simulink model "aero_ground_model"  (R2013b)
settings: Solver=ode23  StartTime=0.0  StopTime=100  FixedStep=0.01  MaxStep=1  RelTol=1e-3
undefined symbols (not defined in the file or in its folder): par
libraries: simulink x12, coeffs x3, lateral_model x3, dspswit3 x1
(part 1 of 2)
settings Model: Creator=goghino  LastModifiedBy=Juraj
settings SolverCC: ZeroCrossAlgorithm=Adaptive  AlgebraicLoopSolver=LineSearch
settings DataIOCC: SignalLoggingSaveFormat=ModelDataLogs
settings DebuggingCC: UnderspecifiedInitializationDetection=Simplified  MultiTaskDSMMsg=warning  MultiTaskCondExecSysMsg=none  SignalLabelMismatchMsg=warning  StrictBusMsg=WarnOnBusTreatedAsVector  NonBusSignalsTreatedAsBus=warning
settings RTWCC: IncludeERTFirstTime=on
settings GRTTargetCC: CodeReplacementLibrary=None  CPPClassGenCompliant=on

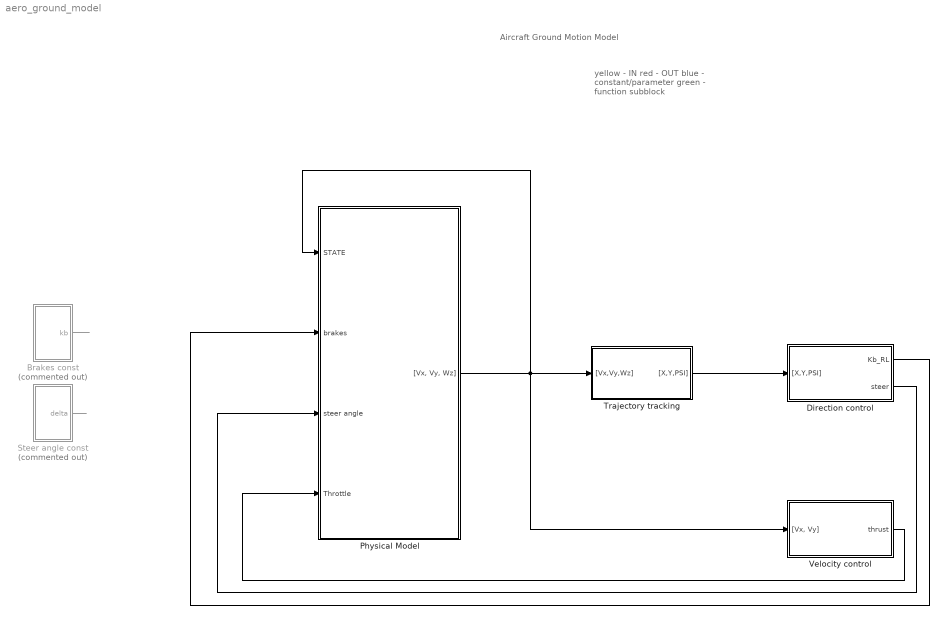
== system aero_ground_model ==
  note: Aircraft Ground Motion Model
  note: yellow - IN
      | red - OUT
      | blue - constant/parameter
      | green - function subblock
  Brakes const : Subsystem  Commented=on
  Direction control : Subsystem
  Physical Model : Subsystem
  Steer angle const : Subsystem  Commented=on
  Trajectory tracking : Subsystem
  Velocity control : Subsystem
  wires:
  Physical Model/1("[Vx, Vy, Wz]") -> Physical Model/1(STATE), Trajectory tracking/1("[Vx,Vy,Wz]"), Velocity control/1("[Vx, Vy]")
  Trajectory tracking/1("[X,Y,PSI]") -> Direction control/1("[X,Y,PSI]")
  Velocity control/1(thrust) -> Physical Model/4(Throttle)
  Direction control/2(steer) -> Physical Model/3(steer angle)
  Direction control/1(Kb_RL) -> Physical Model/2(brakes)
  Steer angle const/1(delta) -> ?
  Brakes const/1(kb) -> ?

== system aero_ground_model/Brakes const ==
  Bus Creator : BusCreator  Inputs=2
  L : Constant  Value=par.kbl
  R : Constant  Value=par.kbr
  kb : Outport
  wires:
  Bus Creator/1 -> kb/1  "Kb"
  R/1 -> Bus Creator/1  "kb_R"
  L/1 -> Bus Creator/2  "kb_L"

== system aero_ground_model/Direction control ==
  "[X,Y,PSI]" : Inport
  Bus Selector : BusSelector  OutputSignals=X,Y,PSI
  Steer PIDs : Subsystem
  Target selector : Subsystem
  To Workspace : ToWorkspace  VariableName=X  SampleTime=-1  SaveFormat=Timeseries
  To Workspace1 : ToWorkspace  VariableName=Y  SampleTime=-1  SaveFormat=Timeseries
  To Workspace2 : ToWorkspace  VariableName=PSI  SampleTime=-1  SaveFormat=Timeseries
  delta heading to target : Subsystem
  Kb_RL : Outport
  steer : Outport  Port=2
  wires:
  Bus Selector/1 -> To Workspace/1  "<X>"
  Bus Selector/2 -> To Workspace1/1  "<Y>"
  Bus Selector/3 -> To Workspace2/1  "<PSI>"
  "[X,Y,PSI]"/1 -> delta heading to target/2(Pos Aero), Target selector/1(Pos Aero), Bus Selector/1
  delta heading to target/1(heading diff) -> Steer PIDs/1("delta heading ")
  Steer PIDs/1(Kb) -> Kb_RL/1
  Steer PIDs/2(steer) -> steer/1
  Target selector/1(Target) -> delta heading to target/1(Pos Target)

== system aero_ground_model/Physical Model ==
  note: Transformation of Forces Acting on Aircraft into State Vector
  note: Physical Model of Aircraft Ground Motion Model
  STATE : Inport
  brakes : Inport  Port=2
  steer angle : Inport  Port=3
  Throttle : Inport  Port=4
  Bus Creator : BusCreator
  Bus Creator1 : BusCreator  Inputs=2
  Bus Creator3 : BusCreator  Inputs=3
  Drag : Subsystem
  Engine model : Subsystem
  Forces to Velocities : Subsystem
  Tire Forces : Subsystem
  X TIRE_FORCES : Scope
      settings: YMin=-140000  YMax=10000  SaveName=ScopeData3
  Y TIRE_FORCES1 : Scope
      settings: YMin=-140000  YMax=10000  SaveName=ScopeData4
  "[Vx, Vy, Wz]" : Outport
  wires:
  Forces to Velocities/2(angular) -> Bus Creator1/2  "Wz"
  Throttle/1 -> Engine model/1(Throttle)
  Bus Creator1/1 -> "[Vx, Vy, Wz]"/1  "STATE"
  steer angle/1 -> Tire Forces/3(delta), Forces to Velocities/8(delta)
  Drag/1(F_xA) -> Forces to Velocities/9(F_xA)
  STATE/1 -> Tire Forces/2(state), Drag/1(STATE), Forces to Velocities/10(STATE)
  Tire Forces/1(F_xN) -> Forces to Velocities/2(F_xN), Bus Creator/1
  Tire Forces/2(F_xL) -> Forces to Velocities/3(F_xL), Bus Creator/2
  Tire Forces/3(F_xR) -> Forces to Velocities/4(F_xR), Bus Creator/3
  Tire Forces/4(F_yN) -> Forces to Velocities/5(F_yN), Bus Creator3/3
  Tire Forces/5(F_yL) -> Bus Creator3/2, Forces to Velocities/6(F_yL)
  Tire Forces/6(F_yR) -> Bus Creator3/1, Forces to Velocities/7(F_yR)
  Forces to Velocities/1(velocity) -> Bus Creator1/1  "[Vx, Vy]"
  brakes/1 -> Tire Forces/4(brakes)
  Bus Creator/1 -> X TIRE_FORCES/1
  Bus Creator3/1 -> Y TIRE_FORCES1/1
  Engine model/1(F_xT) -> Tire Forces/1(thrust), Forces to Velocities/1(F_xT), Bus Creator/4

== system aero_ground_model/Steer angle const ==
  11.5 deg : Constant  Value=0.2
  20 deg : Constant  Value=0.35
  40 deg : Constant  Value=0.7
  5.7 deg : Constant  Value=0.1
  60 deg1 : Constant  Value=1.04
  90 deg : Constant  Value=1.57
  zero : Constant  Value=0
  delta : Outport
  wires:
  11.5 deg/1 -> delta/1

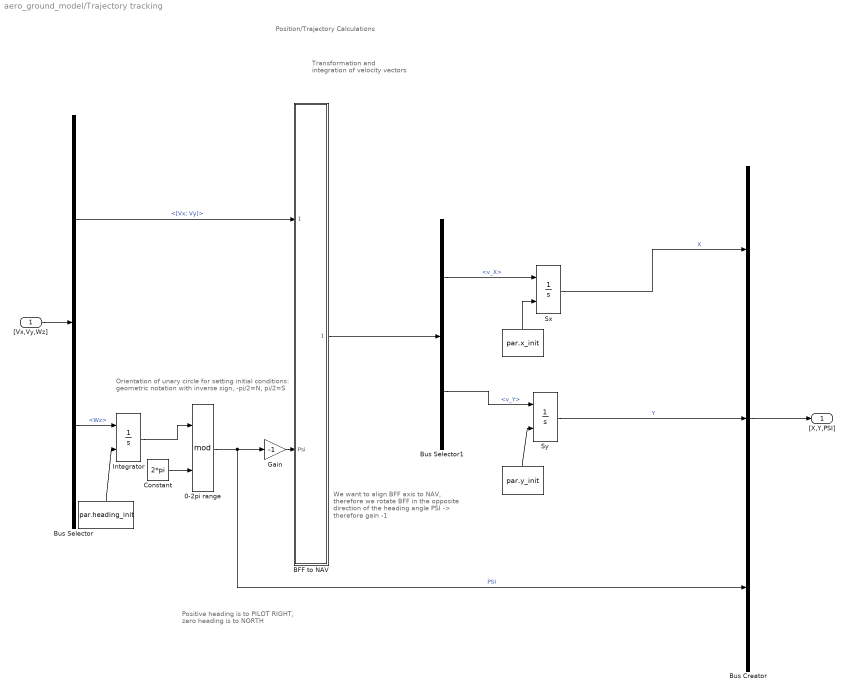
== system aero_ground_model/Trajectory tracking ==
  note: Orientation of unary circle for setting initial conditions:
      | geometric notation with inverse sign, -pi/2=N, pi/2=S
  note: Positive heading is to PILOT RIGHT,
      | zero heading is to NORTH
  note: We want to align BFF axis to NAV,
      | therefore we rotate BFF in the opposite
      | direction of the heading angle PSI ->
      | therefore gain -1
  note: Transformation and integration of velocity vectors
  note: Position/Trajectory Calculations
  "[Vx,Vy,Wz]" : Inport
  " " : Constant  Value=par.heading_init
  "   " : Constant  Value=par.y_init
  "    " : Constant  Value=par.x_init
  0-2pi range : Math  Operator=mod  SaturateOnIntegerOverflow=on
  BFF to NAV : Subsystem
  Bus Creator : BusCreator  Inputs=3
  Bus Selector : BusSelector  OutputSignals=[Vx; Vy],Wz
  Bus Selector1 : BusSelector  OutputSignals=v_X,v_Y
  Constant : Constant  Value=2*pi
  Gain : Gain  Gain=-1
  Integrator : Integrator  InitialConditionSource=external  InitialCondition=pi/2
  Sx : Integrator  InitialConditionSource=external
  Sy : Integrator  InitialConditionSource=external
  "[X,Y,PSI]" : Outport
  wires:
  "[Vx,Vy,Wz]"/1 -> Bus Selector/1
  Bus Selector/1 -> BFF to NAV/1(V_BFF)  "<[Vx; Vy]>"
  BFF to NAV/1(V_NAV) -> Bus Selector1/1
  Bus Selector/2 -> Integrator/1  "<Wz>"
  Bus Selector1/1 -> Sx/1  "<v_X>"
  Bus Selector1/2 -> Sy/1  "<v_Y>"
  Sx/1 -> Bus Creator/1  "X"
  Sy/1 -> Bus Creator/2  "Y"
  Integrator/1 -> 0-2pi range/1
  Constant/1 -> 0-2pi range/2
  0-2pi range/1 -> Bus Creator/3, Gain/1  "PSI"
  Gain/1 -> BFF to NAV/2(Psi)
  Bus Creator/1 -> "[X,Y,PSI]"/1
  " "/1 -> Integrator/2
  "    "/1 -> Sx/2
  "   "/1 -> Sy/2

== system aero_ground_model/Velocity control ==
  note: idea: it takes ±8 sec. to reach full thrust on jet engine,
      | slope = max. trhrust / 8sec falling edge is considered to
      | be twice as fast
  "[Vx, Vy]" : Inport
  Add : Sum  Inputs=-+
  Bus Creator : BusCreator  Inputs=2
  PID Controller : simulink/Continuous/PID Controller  Controller=PID  TimeDomain=Continuous-time  SampleTime=1  IntegratorMethod=Forward Euler  FilterMethod=Forward Euler  Form=Parallel  P=0.2  I=0.05  D=0.8  N=10  InitialConditionSource=internal  InitialConditionForIntegrator=0  InitialConditionForFilter=0  ExternalReset=none  LimitOutput=off  UpperSaturationLimit=inf  LowerSaturationLimit=-inf  LinearizeAsGain=on  AntiWindupMode=none  Kb=1  TrackingMode=off  Kt=1  PParamMin=[]  PParamMax=[]  IParamMin=[]  IParamMax=[]  DParamMin=[]  DParamMax=[]  NParamMin=[]  NParamMax=[]  KbParamMin=[]  KbParamMax=[]  KtParamMin=[]  KtParamMax=[]  POutMin=[]  POutMax=[]  IOutMin=[]  IOutMax=[]  DOutMin=[]  DOutMax=[]  NOutMin=[]  NOutMax=[]  KbOutMin=[]  KbOutMax=[]  KtOutMin=[]  KtOutMax=[]  IntegratorOutMin=[]  IntegratorOutMax=[]  FilterOutMin=[]  FilterOutMax=[]  SumOutMin=[]  SumOutMax=[]  SumI1OutMin=[]  SumI1OutMax=[]  SumI2OutMin=[]  SumI2OutMax=[]  SumI3OutMin=[]  SumI3OutMax=[]  SumDOutMin=[]  SumDOutMax=[]  SaturationOutMin=[]  SaturationOutMax=[]  IntegratorContinuousStateAttributes=''  IntegratorStateMustResolveToSignalObject=off  IntegratorRTWStateStorageClass=Auto  FilterContinuousStateAttributes=''  FilterStateMustResolveToSignalObject=off  FilterRTWStateStorageClass=Auto
  Saturation : Saturate  UpperLimit=1  LowerLimit=0
  Target : Subsystem
  VELOCITY : Scope
      settings: YMin=2  YMax=8
  velocity PID : Scope
      settings: TimeRange=15.53097345132743  YMin=-0.005  YMax=0.105  SaveName=ScopeData10
  |V| : Subsystem
  thrust : Outport
  wires:
  "[Vx, Vy]"/1 -> |V|/1("[vx,vy]")
  |V|/1(V) -> VELOCITY/1, Add/1
  Target/1(V) -> Add/2
  Add/1 -> Bus Creator/1, PID Controller/1  "ref"
  PID Controller/1 -> Saturation/1
  Bus Creator/1 -> velocity PID/1
  Saturation/1 -> Bus Creator/2, thrust/1

== system aero_ground_model/Direction control/Steer PIDs ==
  "delta heading " : Inport
  "BRAKES PID " : Scope
      settings: YMin=-3.5  YMax=3.5  SaveName=ScopeData6
  Bus Creator : BusCreator
  Bus Creator3 : BusCreator  Inputs=2
  Kb_L PID : Subsystem
  Kb_R PID : Subsystem
  steer PID : Subsystem
  Kb : Outport
  steer : Outport  Port=2
  wires:
  Bus Creator3/1 -> Kb/1
  Kb_R PID/1(kb_R) -> Bus Creator/3, Bus Creator3/1  "kb_R"
  Bus Creator/1 -> "BRAKES PID "/1
  Kb_L PID/1(kb_L) -> Bus Creator/4, Bus Creator3/2  "kb_L"
  "delta heading "/1 -> Bus Creator/1, steer PID/1(delta Heading), Kb_R PID/1("delta Heading "), Kb_L PID/1("delta Heading ")
  steer PID/1("steer ") -> steer/1, Bus Creator/2

== system aero_ground_model/Direction control/Target selector ==
  Pos Aero : Inport
  Bus Creator1 : BusCreator  Inputs=2
  Counter : dspswit3/Counter  Direction=Up  CountEvent=Rising edge  CounterSize=32 bits  MaxCount=255  InitialCount=1  Output=Count  HitValue=32  ResetInput=off  SamplesPerFrame=1  Ts=1  CntDtype=double  HitDtype=Logical
  Scope1 : Scope
      settings: YMin=0  YMax=52.5  SaveName=ScopeData11
  Scope2 : Scope
      settings: YMin=0  YMax=52.5  SaveName=ScopeData12
  Targets : Subsystem
  Unit Delay : UnitDelay  SampleTime=-1
  target distance : Subsystem
  target switch distance : simulink/Logic and Bit Operations/Compare To Constant  relop=<  const=par.switch_distance  OutDataTypeStr=uint8
  Target : Outport
  wires:
  Counter/1 -> Bus Creator1/2, Targets/1(idx)
  Pos Aero/1 -> target distance/1(Aero)
  target distance/1(distance) -> Bus Creator1/1, target switch distance/1
  target switch distance/1 -> Counter/1, Scope1/1
  Bus Creator1/1 -> Scope2/1
  Targets/1(Target) -> Unit Delay/1, Target/1
  Unit Delay/1 -> target distance/2(Target)

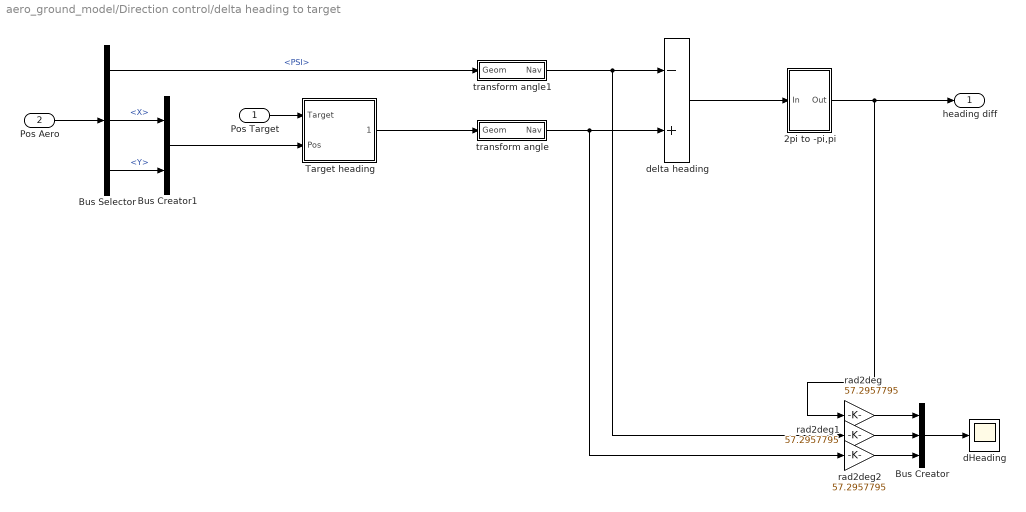
== system aero_ground_model/Direction control/delta heading to target ==
  Pos Target : Inport
  Pos Aero : Inport  Port=2
  2pi to -pi,pi : Subsystem
  Bus Creator : BusCreator  Inputs=3
  Bus Creator1 : BusCreator  Inputs=2
  Bus Selector : BusSelector  OutputSignals=PSI,X,Y
  Target heading : Subsystem
  dHeading : Scope
      settings: TimeRange=25.59999999999991  YMin=-175  YMax=175  SaveName=ScopeData7
  delta heading : Sum  Inputs=-+
  rad2deg : Gain  Gain=57.2957795
  rad2deg1 : Gain  Gain=57.2957795
  rad2deg2 : Gain  Gain=57.2957795
  transform angle : Subsystem
  transform angle1 : Subsystem
  heading diff : Outport
  wires:
  Bus Selector/1 -> transform angle1/1(Geom)  "<PSI>"
  Pos Target/1 -> Target heading/1(Target)
  Bus Creator1/1 -> Target heading/2(Pos)
  Target heading/1(Heading) -> transform angle/1(Geom)
  Bus Creator/1 -> dHeading/1
  rad2deg1/1 -> Bus Creator/2
  rad2deg2/1 -> Bus Creator/3
  transform angle/1(Nav) -> rad2deg2/1, delta heading/2
  rad2deg/1 -> Bus Creator/1
  transform angle1/1(Nav) -> rad2deg1/1, delta heading/1
  2pi to -pi,pi/1(Out) -> heading diff/1, rad2deg/1
  delta heading/1 -> 2pi to -pi,pi/1(In)
  Pos Aero/1 -> Bus Selector/1
  Bus Selector/2 -> Bus Creator1/1  "<X>"
  Bus Selector/3 -> Bus Creator1/2  "<Y>"

== system aero_ground_model/Physical Model/Drag ==
  note: F_xA = 1/2 * RHO * |V|^2 * Sw * Cx
  note: Aerodynamic drag model
  STATE : Inport
  " " : Constant  Value=1/2
  Bus Selector : BusSelector  OutputSignals=[Vx; Vy]
  Cx : Constant  Value=par.Cx
  Product{,1..3} (4 alike) : Product
  RHO : Constant  Value=par.rho
  Sw : Constant  Value=par.Sw
  norm : Subsystem
  sqr : Subsystem
  F_xA : Outport
  wires:
  RHO/1 -> Product/2
  Product/1 -> Product1/1
  Sw/1 -> Product1/2
  Product1/1 -> Product2/1
  Cx/1 -> Product2/2
  Product3/1 -> Product/1
  norm/1(|V|) -> sqr/1(x)
  " "/1 -> Product3/2
  sqr/1(x^2) -> Product3/1
  STATE/1 -> Bus Selector/1
  Bus Selector/1 -> norm/1(V)  "<[Vx; Vy]>"
  Product2/1 -> F_xA/1

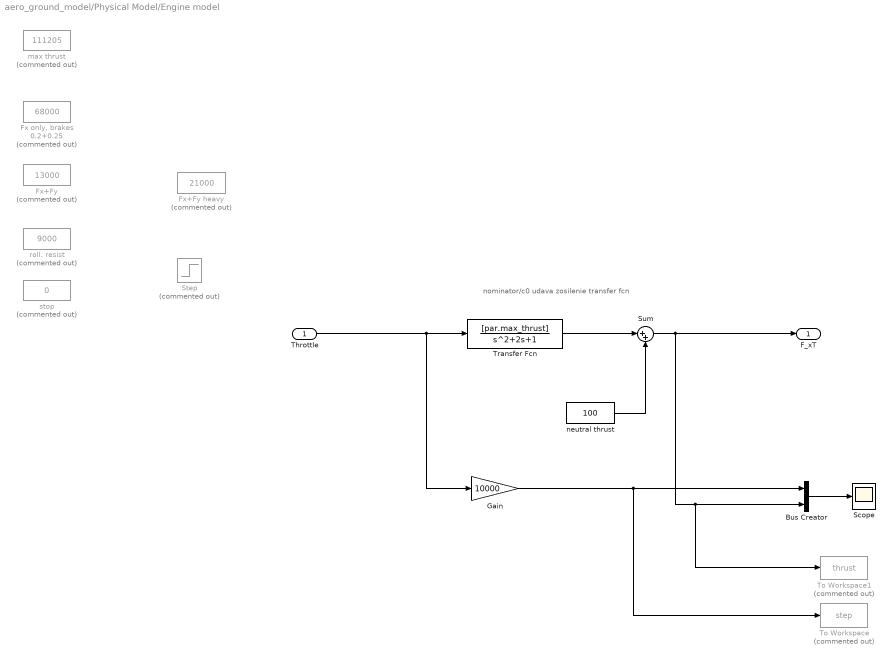
== system aero_ground_model/Physical Model/Engine model ==
  note: nominator/c0 udava zosilenie transfer fcn
  Throttle : Inport
  Bus Creator : BusCreator  Inputs=2
  "Fx only, brakes 0.2+0.25" : Constant  Commented=on  Value=68000
  Fx+Fy : Constant  Commented=on  Value=13000
  Fx+Fy heavy : Constant  Commented=on  Value=21000
  Gain : Gain  Gain=10000
  Scope : Scope
  Step : Step  Commented=on  SampleTime=0
  Sum : Sum  Inputs=|++
  To Workspace : ToWorkspace  Commented=on  VariableName=step  SampleTime=-1  SaveFormat=Timeseries
  To Workspace1 : ToWorkspace  Commented=on  VariableName=thrust  SampleTime=-1  SaveFormat=Timeseries
  Transfer Fcn : TransferFcn  Numerator=[par.max_thrust]
  max thrust : Constant  Commented=on  Value=111205
  neutral thrust : Constant  Value=100
  roll. resist : Constant  Commented=on  Value=9000
  stop : Constant  Commented=on  Value=0
  F_xT : Outport
  wires:
  Transfer Fcn/1 -> Sum/1
  neutral thrust/1 -> Sum/2
  Sum/1 -> F_xT/1, To Workspace1/1, Bus Creator/2
  Bus Creator/1 -> Scope/1
  Throttle/1 -> Gain/1, Transfer Fcn/1
  Gain/1 -> To Workspace/1, Bus Creator/1

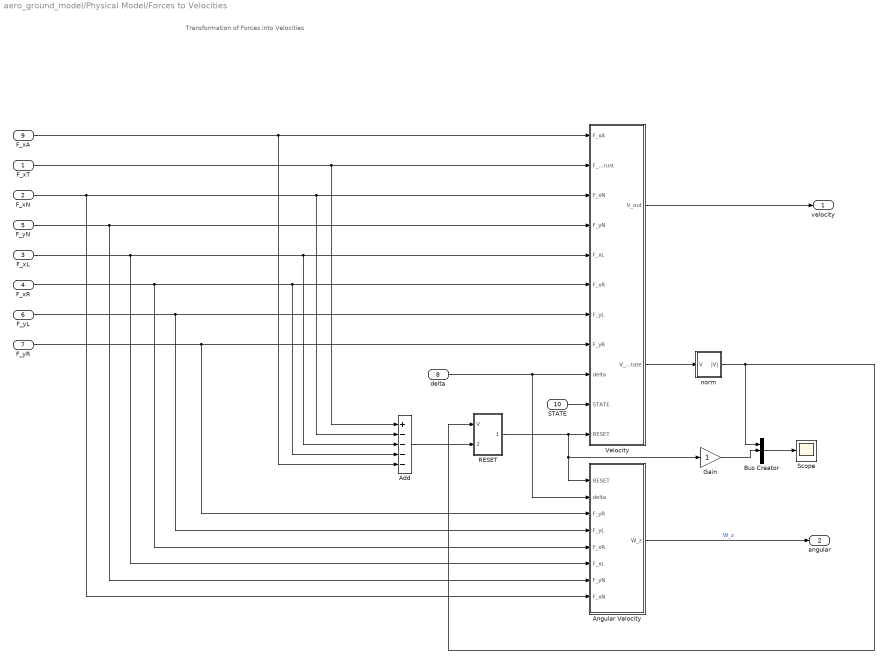
== system aero_ground_model/Physical Model/Forces to Velocities ==
  note: Transformation of Forces into Velocities
  F_xT : Inport
  F_xN : Inport  Port=2
  F_xL : Inport  Port=3
  F_xR : Inport  Port=4
  F_yN : Inport  Port=5
  F_yL : Inport  Port=6
  F_yR : Inport  Port=7
  delta : Inport  Port=8
  F_xA : Inport  Port=9
  STATE : Inport  Port=10
  Add : Sum  Inputs=+----
  Angular Velocity : Subsystem
  Bus Creator : BusCreator  Inputs=3
  Gain : Gain
  RESET : Subsystem
  Scope : Scope
      settings: YMin=0  YMax=8  SaveName=ScopeData5
  Velocity : Subsystem
  norm : Subsystem
  velocity : Outport
  angular : Outport  Port=2
  wires:
  F_xR/1 -> Angular Velocity/5(F_xR), Add/4, Velocity/6(F_xR)
  delta/1 -> Angular Velocity/2(delta), Velocity/9(delta)
  F_xA/1 -> Add/5, Velocity/1(F_xA)
  F_xN/1 -> Angular Velocity/8(F_xN), Add/2, Velocity/3(F_xN)
  F_yL/1 -> Angular Velocity/4(F_yL), Velocity/7(F_yL)
  F_xT/1 -> Velocity/2(F_Thrust), Add/1
  F_yR/1 -> Angular Velocity/3(F_yR), Velocity/8(F_yR)
  F_yN/1 -> Angular Velocity/7(F_yN), Velocity/4(F_yN)
  Velocity/1(V_out) -> velocity/1
  Angular Velocity/1(W_z) -> angular/1  "W_z"
  F_xL/1 -> Angular Velocity/6(F_xL), Add/3, Velocity/5(F_xL)
  STATE/1 -> Velocity/10(STATE)
  RESET/1(RESET) -> Angular Velocity/1(RESET), Gain/1, Velocity/11(RESET)
  norm/1(|V|) -> Bus Creator/1, RESET/1(V)
  Velocity/2(V_out_state) -> norm/1(V)
  Add/1 -> RESET/2(Fx_sum)
  Bus Creator/1 -> Scope/1
  Gain/1 -> Bus Creator/2

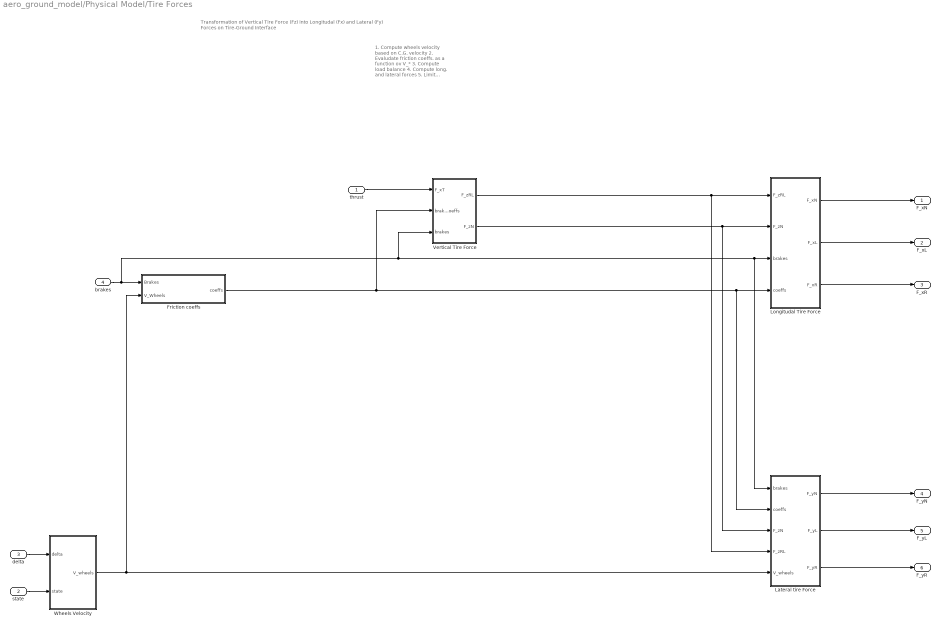
== system aero_ground_model/Physical Model/Tire Forces ==
  note: 1. Compute wheels velocity based on C.G. velocity
      | 2. Evaludate friction coeffs. as a function ov V_*
      | 3. Compute load balance
      | 4. Compute long. and lateral forces
      | 5. Limit output forces at low velocities
  note: Transformation of Vertical Tire Force (Fz) into Longitudal (Fx) and Lateral (Fy) Forces on Tire-Ground Interface
  thrust : Inport
  state : Inport  Port=2
  delta : Inport  Port=3
  brakes : Inport  Port=4
  Friction coeffs : Subsystem
  Lateral tire Force : Subsystem
  Longitudal Tire Force : Subsystem
  Vertical Tire Force : Subsystem
  Wheels Velocity : Subsystem
  F_xN : Outport
  F_xL : Outport  Port=2
  F_xR : Outport  Port=3
  F_yN : Outport  Port=4
  F_yL : Outport  Port=5
  F_yR : Outport  Port=6
  wires:
  Longitudal Tire Force/2(F_xL) -> F_xL/1
  Vertical Tire Force/2(F_zN) -> Lateral tire Force/3(F_zN), Longitudal Tire Force/2(F_zN)
  Vertical Tire Force/1(F_zRL) -> Lateral tire Force/4(F_zRL), Longitudal Tire Force/1(F_zRL)
  Lateral tire Force/1(F_yN) -> F_yN/1
  Lateral tire Force/3(F_yR) -> F_yR/1
  thrust/1 -> Vertical Tire Force/1(F_xT)
  Longitudal Tire Force/3(F_xR) -> F_xR/1
  Lateral tire Force/2(F_yL) -> F_yL/1
  state/1 -> Wheels Velocity/2(state)
  Longitudal Tire Force/1(F_xN) -> F_xN/1
  delta/1 -> Wheels Velocity/1(delta)
  Wheels Velocity/1(V_wheels) -> Friction coeffs/2(V_Wheels), Lateral tire Force/5(V_wheels)
  brakes/1 -> Friction coeffs/1(Brakes), Lateral tire Force/1(brakes), Longitudal Tire Force/3(brakes), Vertical Tire Force/3(brakes)
  Friction coeffs/1(coeffs) -> Lateral tire Force/2(coeffs), Longitudal Tire Force/4(coeffs), Vertical Tire Force/2(braking coeffs)

== system aero_ground_model/Trajectory tracking/BFF to NAV ==
  note: Transformation From BFF into Navigation frame
  V_BFF : Inport
  Psi : Inport  Port=2
  Add : Sum  Inputs=+-
  Add1 : Sum
  Bus Creator : BusCreator  Inputs=2
  Bus Selector : BusSelector  OutputSignals=v_X,v_Y
  Product{,1..3} (4 alike) : Product
  Trigonometric Function : Trigonometry
  Trigonometric Function1 : Trigonometry  Operator=cos
  V_NAV : Outport
  wires:
  V_BFF/1 -> Bus Selector/1
  Bus Selector/1 -> Product2/1, Product/1  "<v_X>"
  Bus Selector/2 -> Product3/1, Product1/1  "<v_Y>"
  Bus Creator/1 -> V_NAV/1
  Psi/1 -> Trigonometric Function1/1, Trigonometric Function/1
  Add/1 -> Bus Creator/1  "v_X"
  Add1/1 -> Bus Creator/2  "v_Y"
  Trigonometric Function1/1 -> Product3/2, Product/2
  Product/1 -> Add/1
  Trigonometric Function/1 -> Product2/2, Product1/2
  Product1/1 -> Add/2
  Product2/1 -> Add1/1
  Product3/1 -> Add1/2

== system aero_ground_model/Velocity control/Target ==
  Target V [m/s] : Constant  Value=par.v_target
  V : Outport
  wires:
  Target V [m/s]/1 -> V/1

== system aero_ground_model/Velocity control/|V| ==
  "[vx,vy]" : Inport
  Add : Sum
  Bus Selector : BusSelector  OutputSignals=[Vx; Vy].v_X,[Vx; Vy].v_Y
  Product : Product
  Product1 : Product
  Sqrt : Sqrt  SaturateOnIntegerOverflow=on
  V : Outport
  wires:
  Add/1 -> Sqrt/1
  Bus Selector/2 -> Product1/2, Product1/1  "<v_Y>"
  "[vx,vy]"/1 -> Bus Selector/1
  Product1/1 -> Add/2
  Product/1 -> Add/1
  Sqrt/1 -> V/1
  Bus Selector/1 -> Product/2, Product/1  "<v_X>"

== system aero_ground_model/Direction control/Steer PIDs/Kb_L PID ==
  note: Differential braking is used for steering only when difference of Heading angle to targed is larger than threshold of max. steering angle
  "delta Heading " : Inport
  Abs : Abs
  Compare To Constant : simulink/Logic and Bit Operations/Compare To Constant  relop=<=  const=-par.max_delta  OutDataTypeStr=boolean
  Multiport Switch : MultiPortSwitch  DataPortOrder=Zero-based contiguous  Inputs=2
  PID Kb_R : simulink/Continuous/PID Controller  Controller=PID  TimeDomain=Continuous-time  SampleTime=1  IntegratorMethod=Forward Euler  FilterMethod=Forward Euler  Form=Parallel  P=10  I=0  D=0  N=100  InitialConditionSource=internal  InitialConditionForIntegrator=0  InitialConditionForFilter=0  ExternalReset=none  LimitOutput=off  UpperSaturationLimit=inf  LowerSaturationLimit=-inf  LinearizeAsGain=on  AntiWindupMode=none  Kb=1  TrackingMode=off  Kt=1  PParamMin=[]  PParamMax=[]  IParamMin=[]  IParamMax=[]  DParamMin=[]  DParamMax=[]  NParamMin=[]  NParamMax=[]  KbParamMin=[]  KbParamMax=[]  KtParamMin=[]  KtParamMax=[]  POutMin=[]  POutMax=[]  IOutMin=[]  IOutMax=[]  DOutMin=[]  DOutMax=[]  NOutMin=[]  NOutMax=[]  KbOutMin=[]  KbOutMax=[]  KtOutMin=[]  KtOutMax=[]  IntegratorOutMin=[]  IntegratorOutMax=[]  FilterOutMin=[]  FilterOutMax=[]  SumOutMin=[]  SumOutMax=[]  SumI1OutMin=[]  SumI1OutMax=[]  SumI2OutMin=[]  SumI2OutMax=[]  SumI3OutMin=[]  SumI3OutMax=[]  SumDOutMin=[]  SumDOutMax=[]  SaturationOutMin=[]  SaturationOutMax=[]  IntegratorContinuousStateAttributes=''  IntegratorStateMustResolveToSignalObject=off  IntegratorRTWStateStorageClass=Auto  FilterContinuousStateAttributes=''  FilterStateMustResolveToSignalObject=off  FilterRTWStateStorageClass=Auto
  Rate limit : RateLimiter  RisingSlewLimit=2  FallingSlewLimit=-2  SampleTimeMode=inherited
  max : Saturate  UpperLimit=1  LowerLimit=0
  "no brakes " : Constant  Value=0
  kb_L : Outport
  wires:
  Compare To Constant/1 -> Multiport Switch/1
  Multiport Switch/1 -> Rate limit/1
  "delta Heading "/1 -> Compare To Constant/1, Abs/1
  PID Kb_R/1 -> max/1
  max/1 -> Multiport Switch/3
  Abs/1 -> PID Kb_R/1
  Rate limit/1 -> kb_L/1  "kb_L"
  "no brakes "/1 -> Multiport Switch/2

== system aero_ground_model/Direction control/Steer PIDs/Kb_R PID ==
  note: Differential braking is used for steering only when difference of Heading angle to targed is larger than threshold of max. steering angle
  "delta Heading " : Inport
  Abs : Abs
  Compare To Constant : simulink/Logic and Bit Operations/Compare To Constant  relop=>=  const=par.max_delta  OutDataTypeStr=boolean
  Multiport Switch : MultiPortSwitch  DataPortOrder=Zero-based contiguous  Inputs=2
  PID Kb_R : simulink/Continuous/PID Controller  Controller=PID  TimeDomain=Continuous-time  SampleTime=1  IntegratorMethod=Forward Euler  FilterMethod=Forward Euler  Form=Parallel  P=10  I=0  D=0  N=100  InitialConditionSource=internal  InitialConditionForIntegrator=0  InitialConditionForFilter=0  ExternalReset=none  LimitOutput=off  UpperSaturationLimit=inf  LowerSaturationLimit=-inf  LinearizeAsGain=on  AntiWindupMode=none  Kb=1  TrackingMode=off  Kt=1  PParamMin=[]  PParamMax=[]  IParamMin=[]  IParamMax=[]  DParamMin=[]  DParamMax=[]  NParamMin=[]  NParamMax=[]  KbParamMin=[]  KbParamMax=[]  KtParamMin=[]  KtParamMax=[]  POutMin=[]  POutMax=[]  IOutMin=[]  IOutMax=[]  DOutMin=[]  DOutMax=[]  NOutMin=[]  NOutMax=[]  KbOutMin=[]  KbOutMax=[]  KtOutMin=[]  KtOutMax=[]  IntegratorOutMin=[]  IntegratorOutMax=[]  FilterOutMin=[]  FilterOutMax=[]  SumOutMin=[]  SumOutMax=[]  SumI1OutMin=[]  SumI1OutMax=[]  SumI2OutMin=[]  SumI2OutMax=[]  SumI3OutMin=[]  SumI3OutMax=[]  SumDOutMin=[]  SumDOutMax=[]  SaturationOutMin=[]  SaturationOutMax=[]  IntegratorContinuousStateAttributes=''  IntegratorStateMustResolveToSignalObject=off  IntegratorRTWStateStorageClass=Auto  FilterContinuousStateAttributes=''  FilterStateMustResolveToSignalObject=off  FilterRTWStateStorageClass=Auto
  Rate limit : RateLimiter  RisingSlewLimit=2  FallingSlewLimit=-2  SampleTimeMode=inherited
  max : Saturate  UpperLimit=1  LowerLimit=0
  "no brakes " : Constant  Value=0
  kb_R : Outport
  wires:
  Compare To Constant/1 -> Multiport Switch/1
  Multiport Switch/1 -> Rate limit/1
  "delta Heading "/1 -> Compare To Constant/1, Abs/1
  PID Kb_R/1 -> max/1
  max/1 -> Multiport Switch/3
  Abs/1 -> PID Kb_R/1
  Rate limit/1 -> kb_R/1  "kb_R"
  "no brakes "/1 -> Multiport Switch/2

== system aero_ground_model/Direction control/Steer PIDs/steer PID ==
  delta Heading : Inport
  PID Controller : simulink/Continuous/PID Controller  Controller=PID  TimeDomain=Continuous-time  SampleTime=1  IntegratorMethod=Forward Euler  FilterMethod=Forward Euler  Form=Parallel  P=1.8  I=0  D=0  N=10  InitialConditionSource=internal  InitialConditionForIntegrator=0  InitialConditionForFilter=0  ExternalReset=none  LimitOutput=off  UpperSaturationLimit=inf  LowerSaturationLimit=-inf  LinearizeAsGain=on  AntiWindupMode=none  Kb=1  TrackingMode=off  Kt=1  PParamMin=[]  PParamMax=[]  IParamMin=[]  IParamMax=[]  DParamMin=[]  DParamMax=[]  NParamMin=[]  NParamMax=[]  KbParamMin=[]  KbParamMax=[]  KtParamMin=[]  KtParamMax=[]  POutMin=[]  POutMax=[]  IOutMin=[]  IOutMax=[]  DOutMin=[]  DOutMax=[]  NOutMin=[]  NOutMax=[]  KbOutMin=[]  KbOutMax=[]  KtOutMin=[]  KtOutMax=[]  IntegratorOutMin=[]  IntegratorOutMax=[]  FilterOutMin=[]  FilterOutMax=[]  SumOutMin=[]  SumOutMax=[]  SumI1OutMin=[]  SumI1OutMax=[]  SumI2OutMin=[]  SumI2OutMax=[]  SumI3OutMin=[]  SumI3OutMax=[]  SumDOutMin=[]  SumDOutMax=[]  SaturationOutMin=[]  SaturationOutMax=[]  IntegratorContinuousStateAttributes=''  IntegratorStateMustResolveToSignalObject=off  IntegratorRTWStateStorageClass=Auto  FilterContinuousStateAttributes=''  FilterStateMustResolveToSignalObject=off  FilterRTWStateStorageClass=Auto
  Rate Limiter : RateLimiter  SampleTimeMode=inherited
  Saturation : Saturate  UpperLimit=par.max_delta  LowerLimit=-par.max_delta
  "steer " : Outport
  wires:
  delta Heading/1 -> PID Controller/1
  PID Controller/1 -> Saturation/1
  Saturation/1 -> Rate Limiter/1  "response"
  Rate Limiter/1 -> "steer "/1

== system aero_ground_model/Direction control/Target selector/Targets ==
  idx : Inport
  Bus Creator : BusCreator  Inputs=2
  Bus Creator1 : BusCreator  Inputs=2
  Bus Creator2 : BusCreator  Inputs=2
  Scope : Scope
      settings: SaveName=ScopeData13
  Scope1 : Scope
      settings: SaveName=ScopeData14
  target selector X : MATLAB Function  TreatAsAtomicUnit=on
  target selector Y : MATLAB Function  TreatAsAtomicUnit=on
  x_targets : Constant  Value=par.x_targets
  y_targets : Constant  Value=par.y_targets
  Target : Outport
  wires:
  y_targets/1 -> target selector Y/1(vals)
  x_targets/1 -> target selector X/1(vals)
  idx/1 -> Bus Creator1/1, Bus Creator2/1, target selector X/2(idx), target selector Y/2(idx)
  target selector X/1(target) -> Bus Creator1/2, Bus Creator/1  "X"
  target selector Y/1(target) -> Bus Creator2/2, Bus Creator/2  "Y"
  Bus Creator/1 -> Target/1
  Bus Creator1/1 -> Scope/1
  Bus Creator2/1 -> Scope1/1

== system aero_ground_model/Direction control/Target selector/target distance ==
  Aero : Inport
  Target : Inport  Port=2
  Add : Sum
  Bus Selector : BusSelector  OutputSignals=X,Y
  Bus Selector1 : BusSelector  OutputSignals=X,Y
  Sqrt : Sqrt  SaturateOnIntegerOverflow=on
  dX : Sum  Inputs=+-
  dY : Sum  Inputs=+-
  dx_sqr : Product
  dy_sqr : Product
  distance : Outport
  wires:
  Bus Selector1/2 -> dY/2  "<Y>"
  Bus Selector/2 -> dY/1  "<Y>"
  dY/1 -> dy_sqr/1, dy_sqr/2
  Bus Selector1/1 -> dX/2  "<X>"
  Target/1 -> Bus Selector/1
  Bus Selector/1 -> dX/1  "<X>"
  Aero/1 -> Bus Selector1/1
  Sqrt/1 -> distance/1
  dX/1 -> dx_sqr/1, dx_sqr/2
  dy_sqr/1 -> Add/1
  dx_sqr/1 -> Add/2
  Add/1 -> Sqrt/1

== system aero_ground_model/Direction control/delta heading to target/2pi to -pi,pi ==
  In : Inport
  " " : Constant  Value=2*pi
  Abs : Abs
  Compare To Constant : simulink/Logic and Bit Operations/Compare To Constant  relop=>  const=pi  OutDataTypeStr=boolean
  Compare To Constant1 : simulink/Logic and Bit Operations/Compare To Constant  relop=>  const=0  OutDataTypeStr=boolean
  Multiport Switch : MultiPortSwitch  DataPortOrder=Zero-based contiguous  Inputs=2
  Sum : Sum  Inputs=|++
  Sum1 : Sum  Inputs=|+-
  "adjunct to 2pi " : MultiPortSwitch  DataPortOrder=Zero-based contiguous  Inputs=2
  Out : Outport
  wires:
  Multiport Switch/1 -> Out/1
  Sum/1 -> "adjunct to 2pi "/2
  Compare To Constant/1 -> Multiport Switch/1
  " "/1 -> Sum/2, Sum1/2
  "adjunct to 2pi "/1 -> Multiport Switch/3
  Compare To Constant1/1 -> "adjunct to 2pi "/1
  Abs/1 -> Compare To Constant/1
  Sum1/1 -> "adjunct to 2pi "/3
  In/1 -> Abs/1, Multiport Switch/2, Compare To Constant1/1, Sum/1, Sum1/1

== system aero_ground_model/Direction control/delta heading to target/Target heading ==
  Target : Inport
  Pos : Inport  Port=2
  Bus Selector : BusSelector  OutputSignals=X,Y
  Bus Selector1 : BusSelector  OutputSignals=X,Y
  Constant : Constant  Commented=on  Value=-1
  Constant1 : Constant  Commented=on
  Display : Display  Commented=on
  Trigonometric Function : Trigonometry  Operator=atan2
  Trigonometric Function1 : Trigonometry  Commented=on  Operator=atan2
  dX : Sum  Inputs=+-
  dY : Sum  Inputs=+-
  "r2d " : Gain  Commented=on  Gain=57.2957795
  Heading : Outport
  wires:
  Bus Selector1/2 -> dY/2  "<Y>"
  Bus Selector/2 -> dY/1  "<Y>"
  dY/1 -> Trigonometric Function/1
  Bus Selector1/1 -> dX/2  "<X>"
  Target/1 -> Bus Selector/1
  Bus Selector/1 -> dX/1  "<X>"
  Pos/1 -> Bus Selector1/1
  Trigonometric Function/1 -> Heading/1
  dX/1 -> Trigonometric Function/2
  Trigonometric Function1/1 -> "r2d "/1
  Constant/1 -> Trigonometric Function1/1
  Constant1/1 -> Trigonometric Function1/2
  "r2d "/1 -> Display/1

== system aero_ground_model/Direction control/delta heading to target/transform angle ==
  note: Conversion from geometric angle to navigational angle
  note: conversion from unary circle
      | to navigational unary circle
      | (shifted zero and clockwise
      | positive direction)
  note: conversion
      | (-pi,pi) 2 (0,2pi)
  Geom : Inport
  " " : Constant  Value=2*pi
  (0,2pi) : Math  Operator=mod  SaturateOnIntegerOverflow=on
  (0,2pi)1 : Math  Operator=mod  SaturateOnIntegerOverflow=on
  Constant : Constant  Value=2*pi
  Constant1 : Constant  Value=pi/2
  Sum : Sum  Inputs=|-+
  Nav : Outport
  wires:
  Geom/1 -> (0,2pi)/1
  " "/1 -> (0,2pi)1/2
  Constant/1 -> (0,2pi)/2
  (0,2pi)/1 -> Sum/1
  Constant1/1 -> Sum/2
  Sum/1 -> (0,2pi)1/1
  (0,2pi)1/1 -> Nav/1

== system aero_ground_model/Direction control/delta heading to target/transform angle1 ==
  note: because of definition of angles
      | during initializing integrator for Wz
  note: Conversion from geometric angle to navigational angle
  note: conversion from unary circle
      | to navigational unary circle
      | (shifted zero and clockwise
      | positive direction)
  note: conversion
      | (-pi,pi) 2 (0,2pi)
  Geom : Inport
  " " : Constant  Value=2*pi
  (0,2pi) : Math  Operator=mod  SaturateOnIntegerOverflow=on
  (0,2pi)1 : Math  Operator=mod  SaturateOnIntegerOverflow=on
  Constant : Constant  Value=2*pi
  Constant1 : Constant  Value=pi/2
  Gain : Gain  Gain=-1
  Sum : Sum  Inputs=|-+
  Nav : Outport
  wires:
  Geom/1 -> Gain/1
  " "/1 -> (0,2pi)1/2
  Constant/1 -> (0,2pi)/2
  (0,2pi)/1 -> Sum/1
  Constant1/1 -> Sum/2
  Sum/1 -> (0,2pi)1/1
  (0,2pi)1/1 -> Nav/1
  Gain/1 -> (0,2pi)/1

== system aero_ground_model/Physical Model/Drag/norm ==
  V : Inport
  Add : Sum
  Bus Selector : BusSelector  OutputSignals=v_X,v_Y
  Sqrt : Sqrt  SaturateOnIntegerOverflow=on
  sqr : Subsystem
  sqr1 : Subsystem
  |V| : Outport
  wires:
  sqr1/1(x^2) -> Add/2
  Sqrt/1 -> |V|/1
  sqr/1(x^2) -> Add/1
  V/1 -> Bus Selector/1
  Bus Selector/1 -> sqr/1(x)  "<v_X>"
  Bus Selector/2 -> sqr1/1(x)  "<v_Y>"
  Add/1 -> Sqrt/1

== system aero_ground_model/Physical Model/Drag/sqr ==
  x : Inport
  Product3 : Product
  x^2 : Outport
  wires:
  x/1 -> Product3/2, Product3/1
  Product3/1 -> x^2/1

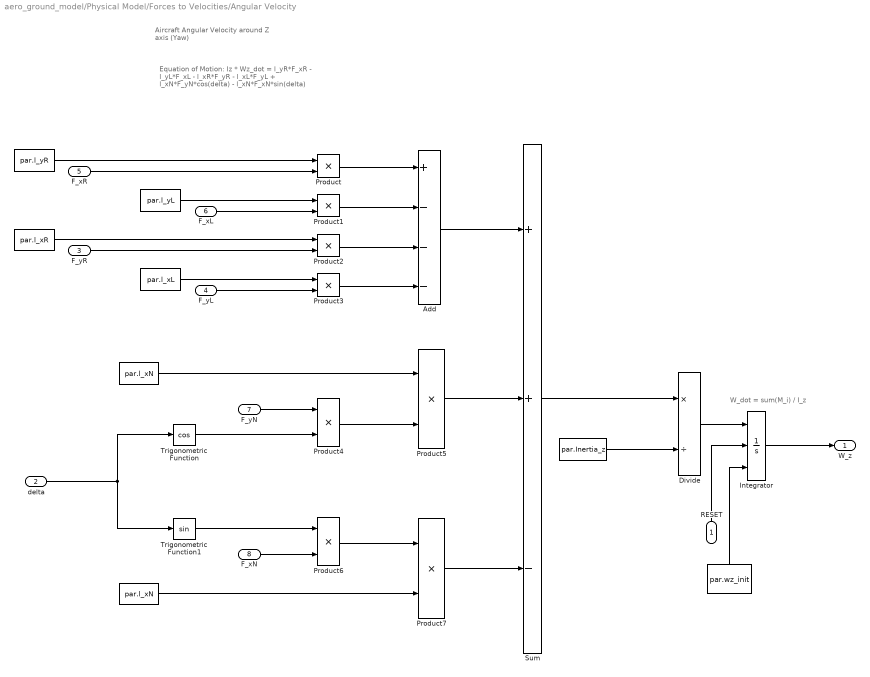
== system aero_ground_model/Physical Model/Forces to Velocities/Angular Velocity ==
  note: Equation of Motion: Iz * Wz_dot = l_yR*F_xR - l_yL*F_xL - l_xR*F_yR - l_xL*F_yL + l_xN*F_yN*cos(delta) - l_xN*F_xN*sin(delta)
  note: Aircraft Angular Velocity around Z axis (Yaw)
  note: W_dot = sum(M_i) / I_z
  RESET : Inport
  delta : Inport  Port=2
  F_yR : Inport  Port=3
  F_yL : Inport  Port=4
  F_xR : Inport  Port=5
  F_xL : Inport  Port=6
  F_yN : Inport  Port=7
  F_xN : Inport  Port=8
  " " : Constant  Value=par.l_yL
  "  " : Constant  Value=par.l_yR
  "   " : Constant  Value=par.l_xR
  "    " : Constant  Value=par.l_xL
  "     " : Constant  Value=par.wz_init
  "       " : Constant  Value=par.Inertia_z
  "        " : Constant  Value=par.l_xN
  "           " : Constant  Value=par.l_xN
  Add : Sum  Inputs=+---
  Divide : Product  Inputs=*/
  Integrator : Integrator  ExternalReset=level hold  InitialConditionSource=external
  Product{,1..7} (8 alike) : Product
  Sum : Sum  Inputs=++-
  Trigonometric Function : Trigonometry  Operator=cos
  Trigonometric Function1 : Trigonometry
  W_z : Outport
  wires:
  Sum/1 -> Divide/1
  Divide/1 -> Integrator/1
  Integrator/1 -> W_z/1
  F_xR/1 -> Product/2
  " "/1 -> Product1/1
  F_xL/1 -> Product1/2
  "   "/1 -> Product2/1
  F_yR/1 -> Product2/2
  "    "/1 -> Product3/1
  F_yL/1 -> Product3/2
  "  "/1 -> Product/1
  "       "/1 -> Divide/2
  delta/1 -> Trigonometric Function/1, Trigonometric Function1/1
  F_yN/1 -> Product4/1
  Trigonometric Function/1 -> Product4/2
  "        "/1 -> Product5/1
  Product4/1 -> Product5/2
  Product5/1 -> Sum/2
  Product7/1 -> Sum/3
  Trigonometric Function1/1 -> Product6/1
  F_xN/1 -> Product6/2
  "           "/1 -> Product7/2
  Product6/1 -> Product7/1
  Product/1 -> Add/1
  Product1/1 -> Add/2
  Product2/1 -> Add/3
  Product3/1 -> Add/4
  Add/1 -> Sum/1
  "     "/1 -> Integrator/3
  RESET/1 -> Integrator/2

== system aero_ground_model/Physical Model/Forces to Velocities/RESET ==
  note: Reset signal becomes: * active when velocity drops below par.min_velo
      | * off when total force reaches certain limit (static friction)
  V : Inport
  Fx_sum : Inport  Port=2
  Compare To Constant : simulink/Logic and Bit Operations/Compare To Constant  relop=<=  const=par.min_velo  OutDataTypeStr=boolean
  Compare To Constant1 : simulink/Logic and Bit Operations/Compare To Constant  relop===  const=0  OutDataTypeStr=boolean
  Compare To Constant2 : simulink/Logic and Bit Operations/Compare To Constant  relop=>=  const=par.min_force  OutDataTypeStr=boolean
  Constant : Constant  Value=0
  Constant1 : Constant
  Constant2 : Constant
  Constant3 : Constant  Value=0
  Constant4 : Constant  Value=0
  Multiport Switch : MultiPortSwitch  DataPortOrder=Zero-based contiguous  Inputs=2
  Multiport Switch1 : MultiPortSwitch  DataPortOrder=Zero-based contiguous  Inputs=2
  Multiport Switch2 : MultiPortSwitch  DataPortOrder=Zero-based contiguous  Inputs=2
  RESET : Outport
  wires:
  Compare To Constant/1 -> Multiport Switch/1
  V/1 -> Compare To Constant/1
  Constant/1 -> Multiport Switch/2
  Constant1/1 -> Multiport Switch/3
  Compare To Constant1/1 -> Multiport Switch1/1
  Multiport Switch/1 -> Compare To Constant1/1
  Multiport Switch1/1 -> RESET/1
  Compare To Constant2/1 -> Multiport Switch2/1
  Fx_sum/1 -> Compare To Constant2/1
  Constant2/1 -> Multiport Switch2/2
  Constant3/1 -> Multiport Switch2/3
  Multiport Switch2/1 -> Multiport Switch1/2
  Constant4/1 -> Multiport Switch1/3

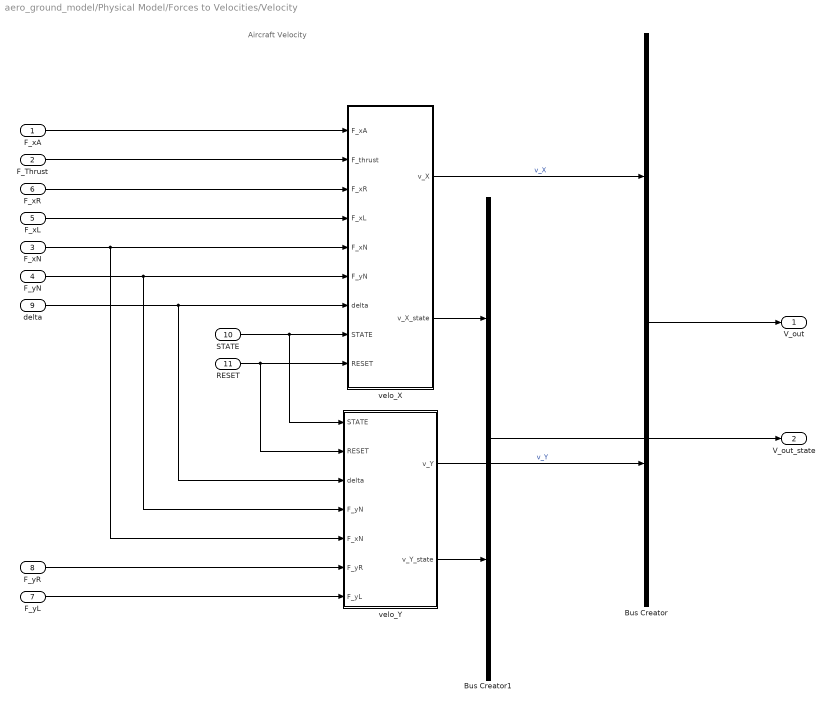
== system aero_ground_model/Physical Model/Forces to Velocities/Velocity ==
  note: Aircraft Velocity
  F_xA : Inport
  F_Thrust : Inport  Port=2
  F_xN : Inport  Port=3
  F_yN : Inport  Port=4
  F_xL : Inport  Port=5
  F_xR : Inport  Port=6
  F_yL : Inport  Port=7
  F_yR : Inport  Port=8
  delta : Inport  Port=9
  STATE : Inport  Port=10
  RESET : Inport  Port=11
  Bus Creator : BusCreator  Inputs=2
  Bus Creator1 : BusCreator  Inputs=2
  velo_X : Subsystem
  velo_Y : Subsystem
  V_out : Outport
  V_out_state : Outport  Port=2
  wires:
  F_xR/1 -> velo_X/3(F_xR)
  F_yL/1 -> velo_Y/7(F_yL)
  F_xL/1 -> velo_X/4(F_xL)
  delta/1 -> velo_X/7(delta), velo_Y/3(delta)
  velo_Y/1(v_Y) -> Bus Creator/2  "v_Y"
  F_xA/1 -> velo_X/1(F_xA)
  F_Thrust/1 -> velo_X/2(F_thrust)
  F_xN/1 -> velo_X/5(F_xN), velo_Y/5(F_xN)
  F_yN/1 -> velo_X/6(F_yN), velo_Y/4(F_yN)
  velo_X/1(v_X) -> Bus Creator/1  "v_X"
  Bus Creator/1 -> V_out/1
  F_yR/1 -> velo_Y/6(F_yR)
  STATE/1 -> velo_X/8(STATE), velo_Y/1(STATE)
  RESET/1 -> velo_X/9(RESET), velo_Y/2(RESET)
  velo_X/2(v_X_state) -> Bus Creator1/1
  velo_Y/2(v_Y_state) -> Bus Creator1/2
  Bus Creator1/1 -> V_out_state/1

== system aero_ground_model/Physical Model/Forces to Velocities/norm ==
  V : Inport
  Add : Sum
  Bus Selector : BusSelector  OutputSignals=signal1,signal2
  Sqrt : Sqrt  SaturateOnIntegerOverflow=on
  sqr : Subsystem
  sqr1 : Subsystem
  |V| : Outport
  wires:
  sqr1/1(x^2) -> Add/2
  Sqrt/1 -> |V|/1
  sqr/1(x^2) -> Add/1
  V/1 -> Bus Selector/1
  Bus Selector/1 -> sqr/1(x)  "<signal1>"
  Bus Selector/2 -> sqr1/1(x)  "<signal2>"
  Add/1 -> Sqrt/1

== system aero_ground_model/Physical Model/Tire Forces/Friction coeffs ==
  note: computed for each wheel separately, since they are function of V and each wheel moves at different speed when turning
  note: Friction coefficients
  Brakes : Inport
  V_Wheels : Inport  Port=2
  Bus Creator : BusCreator  Inputs=3
  Bus Selector : BusSelector  OutputSignals=V_R,V_L,V_N
  Bus Selector1 : BusSelector  OutputSignals=kb_R,kb_L
  Coeffs L : coeffs/Coeffs
  Coeffs N : coeffs/Coeffs
  Coeffs R : coeffs/Coeffs
  No brakes for nose wheel : Constant  Value=0
  coeffs : Outport
  wires:
  V_Wheels/1 -> Bus Selector/1
  Bus Selector/3 -> Coeffs N/2  "<V_N>"
  Bus Selector/2 -> Coeffs L/2  "<V_L>"
  Bus Selector/1 -> Coeffs R/2  "<V_R>"
  Bus Creator/1 -> coeffs/1
  Coeffs R/1 -> Bus Creator/1  "coeffs_R"
  Brakes/1 -> Bus Selector1/1
  Bus Selector1/1 -> Coeffs R/1  "<kb_R>"
  Coeffs L/1 -> Bus Creator/2  "coeffs_L"
  Coeffs N/1 -> Bus Creator/3  "coeffs_N"
  Bus Selector1/2 -> Coeffs L/1  "<kb_L>"
  No brakes for nose wheel/1 -> Coeffs N/1

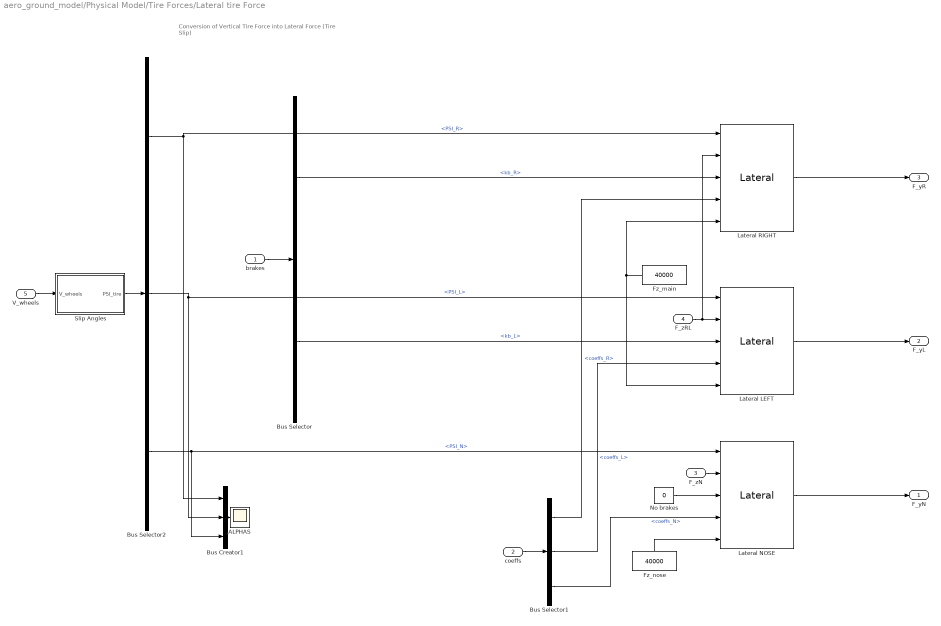
== system aero_ground_model/Physical Model/Tire Forces/Lateral tire Force ==
  note: Conversion of Vertical Tire Force into Lateral Force (Tire Slip)
  brakes : Inport
  coeffs : Inport  Port=2
  F_zN : Inport  Port=3
  F_zRL : Inport  Port=4
  V_wheels : Inport  Port=5
  ALPHAS : Scope
      settings: TimeRange=400  YMin=-0.044  YMax=-0.04125  SaveName=ScopeData2
  Bus Creator1 : BusCreator  Inputs=3
  Bus Selector : BusSelector  OutputSignals=kb_R,kb_L
  Bus Selector1 : BusSelector  OutputSignals=coeffs_R,coeffs_L,coeffs_N
  Bus Selector2 : BusSelector  OutputSignals=PSI_R,PSI_L,PSI_N
  Fz_main : Constant  Value=40000
  Fz_nose : Constant  Value=40000
  Lateral LEFT : lateral_model/Lateral
  Lateral NOSE : lateral_model/Lateral
  Lateral RIGHT : lateral_model/Lateral
  No brakes : Constant  Value=0
  Slip Angles : Subsystem
  F_yN : Outport
  F_yL : Outport  Port=2
  F_yR : Outport  Port=3
  wires:
  F_zN/1 -> Lateral NOSE/2
  V_wheels/1 -> Slip Angles/1(V_wheels)
  Bus Creator1/1 -> ALPHAS/1
  F_zRL/1 -> Lateral RIGHT/2, Lateral LEFT/2
  brakes/1 -> Bus Selector/1
  Bus Selector/2 -> Lateral LEFT/3  "<kb_L>"
  coeffs/1 -> Bus Selector1/1
  Bus Selector/1 -> Lateral RIGHT/3  "<kb_R>"
  Bus Selector1/1 -> Lateral RIGHT/4  "<coeffs_R>"
  Bus Selector1/2 -> Lateral LEFT/4  "<coeffs_L>"
  Bus Selector1/3 -> Lateral NOSE/4  "<coeffs_N>"
  No brakes/1 -> Lateral NOSE/3
  Slip Angles/1(PSI_tire) -> Bus Selector2/1
  Bus Selector2/1 -> Bus Creator1/1, Lateral RIGHT/1  "<PSI_R>"
  Bus Selector2/2 -> Bus Creator1/2, Lateral LEFT/1  "<PSI_L>"
  Bus Selector2/3 -> Lateral NOSE/1, Bus Creator1/3  "<PSI_N>"
  Lateral RIGHT/1 -> F_yR/1
  Lateral NOSE/1 -> F_yN/1
  Lateral LEFT/1 -> F_yL/1
  Fz_main/1 -> Lateral RIGHT/5, Lateral LEFT/5
  Fz_nose/1 -> Lateral NOSE/5

== system aero_ground_model/Physical Model/Tire Forces/Longitudal Tire Force ==
  note: Assuming that F_zR == F_zL
  note: Conversion of Vertical Tire Force into Longitudal Force (Resistance Force)
  F_zRL : Inport
  F_zN : Inport  Port=2
  brakes : Inport  Port=3
  coeffs : Inport  Port=4
  Braking : Subsystem
  Rolling Resistance : Subsystem
  Sum : Sum  Inputs=|++
  Sum1 : Sum  Inputs=|++
  F_xN : Outport
  F_xL : Outport  Port=2
  F_xR : Outport  Port=3
  wires:
  F_zRL/1 -> Braking/1(F_zRL), Rolling Resistance/1(F_zRL)
  F_zN/1 -> Rolling Resistance/2(F_zN)
  Rolling Resistance/1(F_xN) -> F_xN/1
  Sum/1 -> F_xL/1
  Rolling Resistance/2(F_xL) -> Sum/1
  Braking/1(F_xL) -> Sum/2
  Sum1/1 -> F_xR/1
  Braking/2(F_xR) -> Sum1/2
  Rolling Resistance/3(F_xR) -> Sum1/1
  coeffs/1 -> Braking/2(environ), Rolling Resistance/3(coeffs)
  brakes/1 -> Braking/3(brakes)

== system aero_ground_model/Physical Model/Tire Forces/Vertical Tire Force ==
  note: 1. F_zN + F_zR + F_zL = Fg, assuming F_zR==F_zL
      |
      | 2. F_zN*(l_xN - mu_r*l_zN) + 2*F_zR*(-l_xR - mu_r*l_zR) = -l_zT * F_xT
  note: Tire Vertical Forces
  F_xT : Inport
  braking coeffs : Inport  Port=2
  brakes : Inport  Port=3
  " " : Constant  Value=par.weight
  "  " : Constant  Value=par.g
  Add : Sum  Inputs=-+
  Bus Creator : BusCreator  Inputs=2
  Constant : Constant  Value=2
  Product : Product
  Scope : Scope
      settings: SaveName=ScopeData9
  Solver : Subsystem
  m*g : Product
  F_zRL : Outport
  F_zN : Outport  Port=2
  wires:
  Constant/1 -> Product/2
  Solver/1(F_zRL) -> Product/1, Bus Creator/1, F_zRL/1
  Product/1 -> Add/1
  Add/1 -> F_zN/1, Bus Creator/2
  m*g/1 -> Add/2
  " "/1 -> m*g/1
  "  "/1 -> m*g/2
  F_xT/1 -> Solver/1(F_xT)
  brakes/1 -> Solver/2(brakes)
  braking coeffs/1 -> Solver/3(braking coeffs)
  Bus Creator/1 -> Scope/1

== system aero_ground_model/Physical Model/Tire Forces/Wheels Velocity ==
  delta : Inport
  state : Inport  Port=2
  Bus Creator : BusCreator  Inputs=3
  Velocity_L : Subsystem
  Velocity_N : Subsystem
  Velocity_R : Subsystem
  V_wheels : Outport
  wires:
  Velocity_L/1(V_L) -> Bus Creator/2  "V_L"
  Velocity_N/1(V_N) -> Bus Creator/3  "V_N"
  state/1 -> Velocity_N/1(STATE), Velocity_L/1(STATE), Velocity_R/1(STATE)
  delta/1 -> Velocity_N/2(delta)
  Velocity_R/1(V_R) -> Bus Creator/1  "V_R"
  Bus Creator/1 -> V_wheels/1

== system aero_ground_model/Physical Model/Drag/norm/sqr ==
  x : Inport
  Product3 : Product
  x^2 : Outport
  wires:
  x/1 -> Product3/2, Product3/1
  Product3/1 -> x^2/1

== system aero_ground_model/Physical Model/Drag/norm/sqr1 ==
  x : Inport
  Product3 : Product
  x^2 : Outport
  wires:
  x/1 -> Product3/2, Product3/1
  Product3/1 -> x^2/1

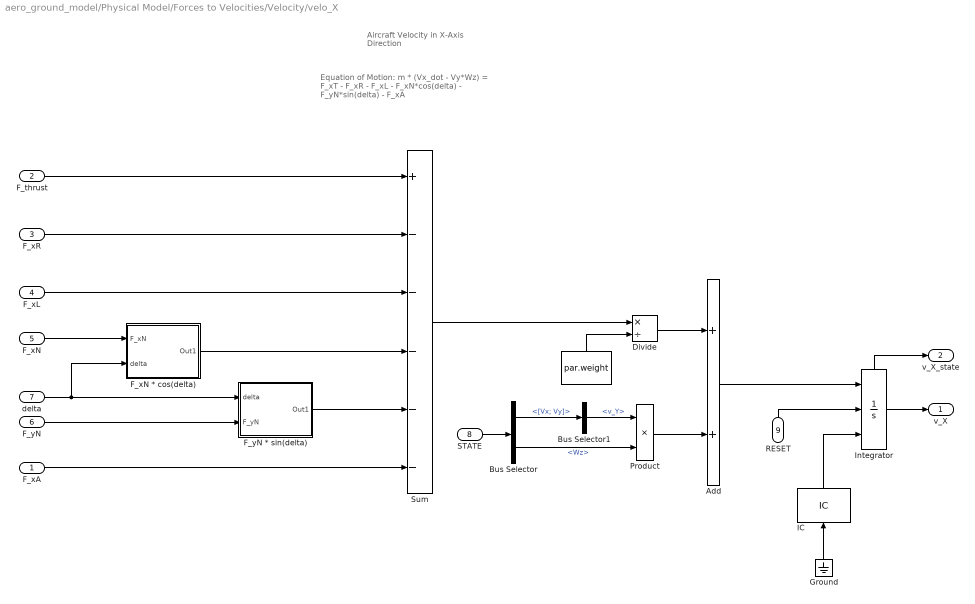
== system aero_ground_model/Physical Model/Forces to Velocities/Velocity/velo_X ==
  note: Equation of Motion: m * (Vx_dot - Vy*Wz) = F_xT - F_xR - F_xL - F_xN*cos(delta) - F_yN*sin(delta) - F_xA
  note: Aircraft Velocity in X-Axis Direction
  F_xA : Inport
  F_thrust : Inport  Port=2
  F_xR : Inport  Port=3
  F_xL : Inport  Port=4
  F_xN : Inport  Port=5
  F_yN : Inport  Port=6
  delta : Inport  Port=7
  STATE : Inport  Port=8
  RESET : Inport  Port=9
  " " : Constant  Value=par.weight
  Add : Sum
  Bus Selector : BusSelector  OutputSignals=[Vx; Vy],Wz
  Bus Selector1 : BusSelector  OutputSignals=v_Y
  Divide : Product  Inputs=*/
  F_xN * cos(delta) : Subsystem
  F_yN * sin(delta) : Subsystem
  Ground : Ground
  IC : InitialCondition  Value=par.vx_init
  Integrator : Integrator  ExternalReset=level hold  InitialConditionSource=external  ShowStatePort=on
  Product : Product
  Sum : Sum  Inputs=+-----
  v_X : Outport
  v_X_state : Outport  Port=2
  wires:
  " "/1 -> Divide/2
  delta/1 -> F_yN * sin(delta)/1(delta), F_xN * cos(delta)/2(delta)
  Integrator/1 -> v_X/1
  F_xN * cos(delta)/1(Out1) -> Sum/4
  F_yN * sin(delta)/1(Out1) -> Sum/5
  F_xR/1 -> Sum/2
  F_xL/1 -> Sum/3
  F_xN/1 -> F_xN * cos(delta)/1(F_xN)
  F_xA/1 -> Sum/6
  F_thrust/1 -> Sum/1
  Sum/1 -> Divide/1
  Divide/1 -> Add/1
  Add/1 -> Integrator/1
  STATE/1 -> Bus Selector/1
  Bus Selector/1 -> Bus Selector1/1  "<[Vx; Vy]>"
  Bus Selector1/1 -> Product/1  "<v_Y>"
  Bus Selector/2 -> Product/2  "<Wz>"
  Product/1 -> Add/2
  F_yN/1 -> F_yN * sin(delta)/2(F_yN)
  RESET/1 -> Integrator/2
  Integrator/State -> v_X_state/1
  IC/1 -> Integrator/3
  Ground/1 -> IC/1

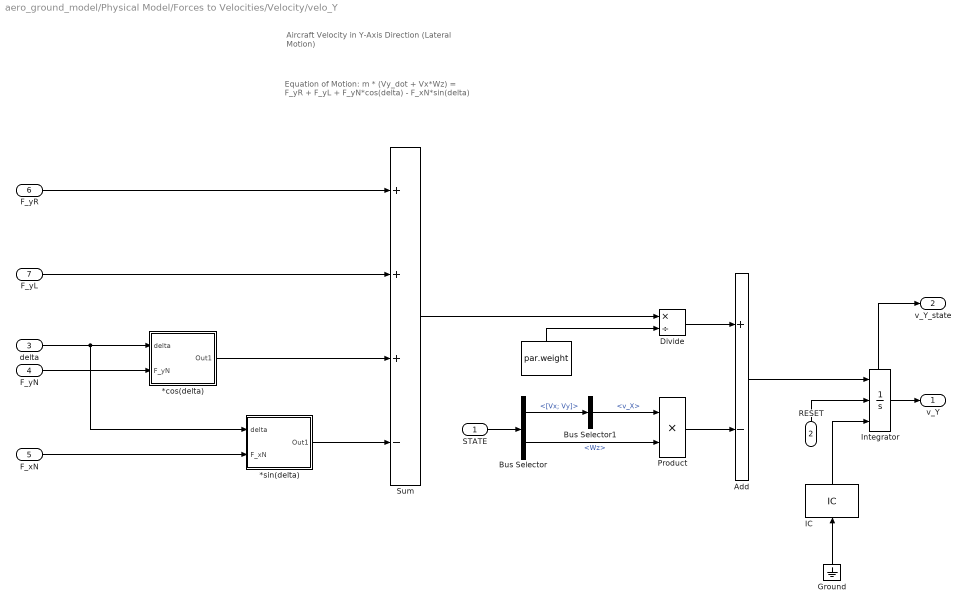
== system aero_ground_model/Physical Model/Forces to Velocities/Velocity/velo_Y ==
  note: Equation of Motion: m * (Vy_dot + Vx*Wz) = F_yR + F_yL + F_yN*cos(delta) - F_xN*sin(delta)
  note: Aircraft Velocity in Y-Axis Direction (Lateral Motion)
  STATE : Inport
  RESET : Inport  Port=2
  delta : Inport  Port=3
  F_yN : Inport  Port=4
  F_xN : Inport  Port=5
  F_yR : Inport  Port=6
  F_yL : Inport  Port=7
  " " : Constant  Value=par.weight
  *cos(delta) : Subsystem
  *sin(delta) : Subsystem
  Add : Sum  Inputs=+-
  Bus Selector : BusSelector  OutputSignals=[Vx; Vy],Wz
  Bus Selector1 : BusSelector  OutputSignals=v_X
  Divide : Product  Inputs=*/
  Ground : Ground
  IC : InitialCondition  Value=par.vy_init
  Integrator : Integrator  ExternalReset=level hold  InitialConditionSource=external  ShowStatePort=on
  Product : Product
  Sum : Sum  Inputs=+++-
  v_Y : Outport
  v_Y_state : Outport  Port=2
  wires:
  delta/1 -> *sin(delta)/1(delta), *cos(delta)/1(delta)
  Integrator/1 -> v_Y/1
  *cos(delta)/1(Out1) -> Sum/3
  *sin(delta)/1(Out1) -> Sum/4
  F_yR/1 -> Sum/1
  F_yL/1 -> Sum/2
  F_yN/1 -> *cos(delta)/2(F_yN)
  F_xN/1 -> *sin(delta)/2(F_xN)
  " "/1 -> Divide/2
  Sum/1 -> Divide/1
  STATE/1 -> Bus Selector/1
  Divide/1 -> Add/1
  Add/1 -> Integrator/1
  Bus Selector/1 -> Bus Selector1/1  "<[Vx; Vy]>"
  Bus Selector1/1 -> Product/1  "<v_X>"
  Bus Selector/2 -> Product/2  "<Wz>"
  Product/1 -> Add/2
  RESET/1 -> Integrator/2
  Integrator/State -> v_Y_state/1
  IC/1 -> Integrator/3
  Ground/1 -> IC/1

== system aero_ground_model/Physical Model/Forces to Velocities/norm/sqr ==
  x : Inport
  Product3 : Product
  x^2 : Outport
  wires:
  x/1 -> Product3/2, Product3/1
  Product3/1 -> x^2/1

== system aero_ground_model/Physical Model/Forces to Velocities/norm/sqr1 ==
  x : Inport
  Product3 : Product
  x^2 : Outport
  wires:
  x/1 -> Product3/2, Product3/1
  Product3/1 -> x^2/1

== system aero_ground_model/Physical Model/Tire Forces/Lateral tire Force/Slip Angles ==
  note: Tire Slip Angle (Velocity Vector x Tire Axis)
  V_wheels : Inport
  Bus Creator : BusCreator  Inputs=3
  Bus Selector : BusSelector  OutputSignals=V_R,V_L,V_N
  arctan(V_L) : Subsystem
  arctan(V_N) : Subsystem
  arctan(V_R) : Subsystem
  PSI_tire : Outport
  wires:
  arctan(V_R)/1(atan(V)) -> Bus Creator/1  "PSI_R"
  arctan(V_L)/1(atan(V)) -> Bus Creator/2  "PSI_L"
  V_wheels/1 -> Bus Selector/1
  Bus Selector/1 -> arctan(V_R)/1(V)  "<V_R>"
  Bus Selector/2 -> arctan(V_L)/1(V)  "<V_L>"
  Bus Selector/3 -> arctan(V_N)/1(V)  "<V_N>"
  arctan(V_N)/1(atan(V)) -> Bus Creator/3  "PSI_N"
  Bus Creator/1 -> PSI_tire/1

== system aero_ground_model/Physical Model/Tire Forces/Longitudal Tire Force/Braking ==
  F_zRL : Inport
  environ : Inport  Port=2
  brakes : Inport  Port=3
  Bus Selector : BusSelector  OutputSignals=kb_R,kb_L
  L brake : Subsystem
  R brake : Subsystem
  F_xL : Outport
  F_xR : Outport  Port=2
  wires:
  F_zRL/1 -> L brake/1(F_zRL), R brake/2(F_zRL)
  environ/1 -> L brake/2(environ), R brake/3(environ)
  R brake/1(F_xR) -> F_xR/1
  L brake/1(F_xL) -> F_xL/1
  brakes/1 -> Bus Selector/1
  Bus Selector/1 -> R brake/1(brakes)  "<kb_R>"
  Bus Selector/2 -> L brake/3(brakes)  "<kb_L>"

== system aero_ground_model/Physical Model/Tire Forces/Longitudal Tire Force/Rolling Resistance ==
  F_zRL : Inport
  F_zN : Inport  Port=2
  coeffs : Inport  Port=3
  Bus Selector1 : BusSelector  OutputSignals=coeffs_L,coeffs_R,coeffs_N
  Resist_L : Subsystem
  Resist_N : Subsystem
  Resist_R : Subsystem
  F_xN : Outport
  F_xL : Outport  Port=2
  F_xR : Outport  Port=3
  wires:
  F_zN/1 -> Resist_N/1(F_zN)
  F_zRL/1 -> Resist_R/1(F_zR), Resist_L/2(F_zL)
  Resist_L/1(F_xL) -> F_xL/1
  Resist_N/1(F_xN) -> F_xN/1
  Resist_R/1(F_xR) -> F_xR/1
  coeffs/1 -> Bus Selector1/1
  Bus Selector1/1 -> Resist_L/1(coeffs)  "<coeffs_L>"
  Bus Selector1/2 -> Resist_R/2(coeffs)  "<coeffs_R>"
  Bus Selector1/3 -> Resist_N/2(coeffs)  "<coeffs_N>"

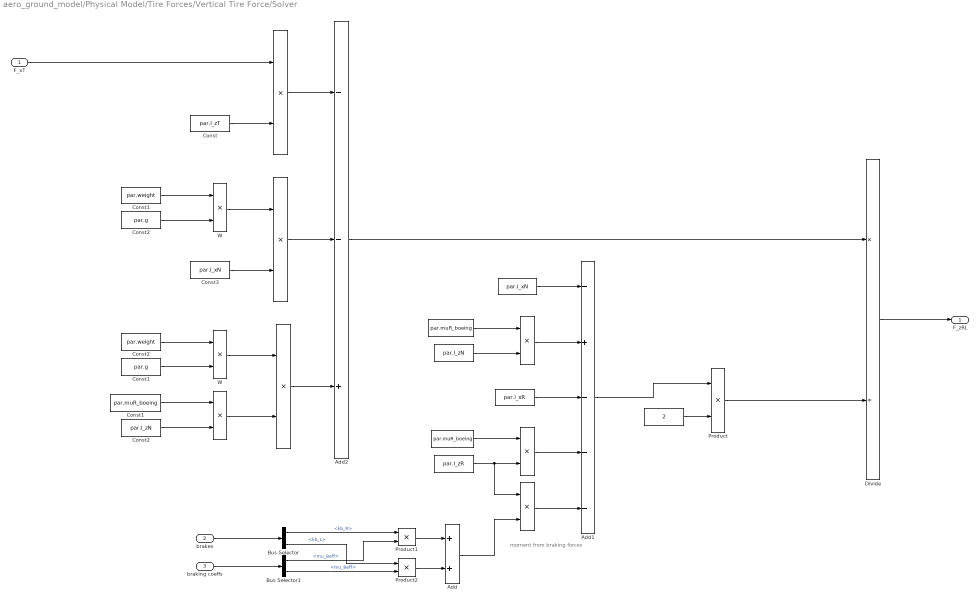
== system aero_ground_model/Physical Model/Tire Forces/Vertical Tire Force/Solver ==
  note: moment from
      | braking forces
  F_xT : Inport
  brakes : Inport  Port=2
  braking coeffs : Inport  Port=3
  "      " : Constant  Value=par.l_xN
  "           " : Product
  "            " : Constant  Value=par.muR_boeing
  "                  " : Constant  Value=2
  "                     " : Constant  Value=par.l_zN
  "                         " : Constant  Value=par.l_zR
  "                          " : Product
  "                             " : Constant  Value=par.l_xR
  "                              " : Product
  "                                  " : Product
  "                                     " : Product
  "                                        " : Constant  Value=par.muR_boeing
  "                                             " : Product
  "                                              " : Product
  "  Const1" : Constant  Value=par.g
  "  Const2" : Constant  Value=par.g
  " Const1" : Constant  Value=par.weight
  " Const2" : Constant  Value=par.weight
  Add : Sum
  Add1 : Sum  Inputs=-+---
  Add2 : Sum  Inputs=--+
  Bus Selector : BusSelector  OutputSignals=kb_R,kb_L
  Bus Selector1 : BusSelector  OutputSignals=coeffs_R.mu_Beff,coeffs_L.mu_Beff
  Const : Constant  Value=par.l_zT
  Const1 : Constant  Value=par.muR_boeing
  Const2 : Constant  Value=par.l_zN
  Const3 : Constant  Value=par.l_xN
  Divide : Product  Inputs=*/
  Product : Product
  Product1 : Product
  Product2 : Product
  W : Product
  "W " : Product
  F_zRL : Outport
  wires:
  F_xT/1 -> "           "/1
  "  Const2"/1 -> W/2
  "                     "/1 -> "                          "/2
  "                              "/1 -> Add2/2
  " Const1"/1 -> W/1
  "                                        "/1 -> "                                  "/1
  "            "/1 -> "                          "/1
  "                          "/1 -> Add1/2
  Const/1 -> "           "/2
  "  Const1"/1 -> "W "/2
  Const1/1 -> "                                              "/1
  "W "/1 -> "                                             "/1
  "                             "/1 -> Add1/3
  "                                  "/1 -> Add1/4
  Const2/1 -> "                                              "/2
  Add1/1 -> Product/1
  "      "/1 -> Add1/1
  W/1 -> "                              "/1
  "           "/1 -> Add2/1
  " Const2"/1 -> "W "/1
  "                                             "/1 -> Add2/3
  "                                              "/1 -> "                                             "/2
  Const3/1 -> "                              "/2
  Divide/1 -> F_zRL/1
  Add2/1 -> Divide/1
  "                  "/1 -> Product/2
  Product/1 -> Divide/2
  brakes/1 -> Bus Selector/1
  braking coeffs/1 -> Bus Selector1/1
  Bus Selector/1 -> Product1/1  "<kb_R>"
  Bus Selector/2 -> Product2/1  "<kb_L>"
  Bus Selector1/1 -> Product1/2  "<mu_Beff>"
  Bus Selector1/2 -> Product2/2  "<mu_Beff>"
  Product1/1 -> Add/1
  Product2/1 -> Add/2
  "                                     "/1 -> Add1/5
  "                         "/1 -> "                                     "/1, "                                  "/2
  Add/1 -> "                                     "/2
